simulink library "ssreuselib"  (R2022b)
settings: Solver=VariableStepAuto  StartTime=0.0  StopTime=10.0  RelTol=1e-3
undefined symbols (not defined in the file): T1Break, T1Data
settings Model: Creator=amyyang  LastModifiedBy=amyyang

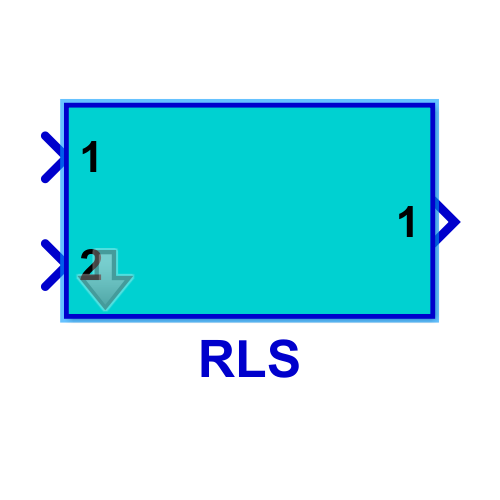
[thumbnail: Simulink's stored preview of the top-level diagram]
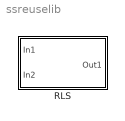
== system ssreuselib ==
  RLS : Subsystem  TreatAsAtomicUnit=on  RTWFcnName=myfun_$C  RTWFileName=myfile  mask(SSDemo){x=T1Break, y=T1Data}
      mask prompts: x "Break points (X data):"; y "Output values (Y data):"
      mask help: Example to show code reuse. This example has two parameters for a lookup table.
      settings: RTWFcnNameOpts=User specified

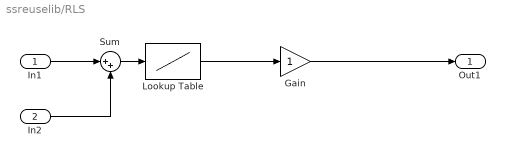
== system ssreuselib/RLS ==
  In1 : Inport  OutDataTypeStr=double
  In2 : Inport  Port=2  OutDataTypeStr=double
  Gain : Gain
  Lookup Table : Lookup_n-D  NumberOfTableDimensions=1  BreakpointsForDimension1=x  Table=y
  Sum : Sum  Inputs=|++
  Out1 : Outport  OutDataTypeStr=double  VectorParamsAs1DForOutWhenUnconnected=off
  wires:
  Sum/1 -> Lookup Table/1
  In2/1 -> Sum/2
  In1/1 -> Sum/1
  Lookup Table/1 -> Gain/1
  Gain/1 -> Out1/1
